simulink model "ON_OFF"  (Simulink 7.7)
settings: Solver=ode3  StartTime=0.0  StopTime=10.0  FixedStep=0.1  RelTol=1e-3
settings Model: Creator=danwheeler  LastModifiedBy=danwheeler
settings DataIOCC: ExternalInput=[t, u1, u2, u3, u4]  LoadExternalInput=on  SaveFinalState=on  SaveCompleteFinalSimState=on

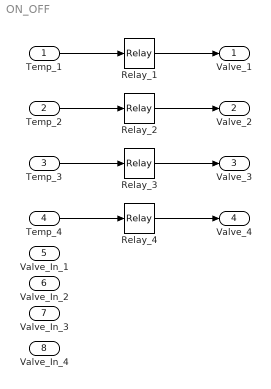
== system ON_OFF ==
  Temp_1 : Inport
  Temp_2 : Inport  Port=2
  Temp_3 : Inport  Port=3
  Temp_4 : Inport  Port=4
  Valve_In_1 : Inport  Port=5
  Valve_In_2 : Inport  Port=6
  Valve_In_3 : Inport  Port=7
  Valve_In_4 : Inport  Port=8
  Relay_1 : Relay  OnSwitchValue=22  OffSwitchValue=20  OnOutputValue=90  OffOutputValue=9
  Relay_2 : Relay  OnSwitchValue=22  OffSwitchValue=20  OnOutputValue=90
  Relay_3 : Relay  OnSwitchValue=22  OffSwitchValue=20  OnOutputValue=90
  Relay_4 : Relay  OnSwitchValue=22  OffSwitchValue=20  OnOutputValue=90
  Valve_1 : Outport
  Valve_2 : Outport  Port=2
  Valve_3 : Outport  Port=3
  Valve_4 : Outport  Port=4
  wires:
  Temp_1/1 -> Relay_1/1
  Relay_1/1 -> Valve_1/1
  Temp_2/1 -> Relay_2/1
  Relay_2/1 -> Valve_2/1
  Temp_3/1 -> Relay_3/1
  Relay_3/1 -> Valve_3/1
  Temp_4/1 -> Relay_4/1
  Relay_4/1 -> Valve_4/1
